simulink model "windEmulatorStep4"  (R2022b)
settings: Solver=ode4  StartTime=0.0  StopTime=inf  FixedStep=Ts  RelTol=1e-3
values from neighbouring files (symbols this model uses):
  A = 1.0    (= 1)    [initStep4.m]
  absEncoderCountsToRad = 1/2^20*2*pi    (= 5.99211245268e-06)    [initStep4.m]
  acs800DcBusVoltsScaling = 1    [initStep4.m]
  acs800FreqScaling = 1/100    (= 0.01)    [initStep4.m]
  acs800PowerScaling = Gen_PowerScaling    (= 14.9109)    [initStep4.m]
  acs800SpeedNomEng = 1500    [initStep4.m]
  acs800SpeedNomFb = 20000    [initStep4.m]
  acs800SpeedScaling = 1500/20000    (= 0.075)    [initStep4.m]
  acs800TempScaling = 1/10    (= 0.1)    [initStep4.m]
  acs800TorqueNomEng = 100    [initStep4.m]
  acs800TorqueNomFb = 10000    [initStep4.m]
  acs800TorqueScaling = acs800TorqueRating/10000    (= 0.008035933)    [initStep4.m]
  acs880FreqScaling = 60/20000    (= 0.003)    [initStep4.m]
  acs880MotorCurrentScaling = 100/10000    (= 0.01)    [initStep4.m]
  acs880MotorVoltsScaling = 1    [initStep4.m]
  acs880PowerScaling = 100*hp2W/10000    (= 7.457)    [initStep4.m]
  acs880RatedTorque = 80.494    [initStep4.m]
  acs880RateLimFalling = -10000    [initStep4.m]
  acs880RateLimRising = 10000    [initStep4.m]
  acs880SetpointLimLower = -0.975*acs880RatedTorque    (= -78.48165)    [initStep4.m]
  acs880SetpointLimUpper = 0.975*acs880RatedTorque    (= 78.48165)    [initStep4.m]
  acs880SpeedPILimLo = -0.975*acs880RatedTorque    (= -78.48165)    [initStep4.m]
  acs880SpeedPILimUp = 0.975*acs880RatedTorque    (= 78.48165)    [initStep4.m]
  acs880SpeedScaling = 2000/20000    (= 0.1)    [initStep4.m]
  acs880TorqueFieldbusScale = 10000    [initStep4.m]
  acs880TorqueScaling = acs880RatedTorque/acs880TorqueFieldbusScale    (= 0.0080494)    [initStep4.m]
  acs880TorqueSetpointScaling = 100    [initStep4.m]
  bar2pa = 1e5    (= 100000)    [initStep4.m]
  belowMinPGain = 1/200    (= 0.005)    [initStep4.m]
  ctrlModeTorque = logical(true)    [initStep4.m]
  deadBandController = boolean(true)    [initStep4.m]
  deadbandTorqueSlewRate = 300    [initStep4.m]
  Dm_max = 40    [initStep4.m]
  EffMechMax = 0.93    [initStep4.m]
  EffMechMin = 0.79    [initStep4.m]
  FactorEff = psi2pa*cc2m3*(1/rev2rad)    (= 0.00109733470463)    [initStep4.m]
  fromFileSpeedSlewRate = 250    [initStep4.m]
  fromFileTorqueSlewRate = 25    [initStep4.m]
  futekTorqueScale = -1/(2^31)*10/5*100    (= -9.31322574615e-08)    [initStep4.m]
  genMaxTorque = 0.975*acs880RatedTorque    (= 78.48165)    [initStep4.m]
  hbmCtScale = 1/1.5    (= 0.666666666667)    [initStep4.m]
  lpm2m3ps = 1/m3ps2lpm    (= 1.66666666667e-05)    [initStep4.m]
  minPressureRef_psi = 1000    [initStep4.m]
  minTorqueRef_Nm = (minPressureRef_psi*psi2pa)*(Dm_max*cc2m3*(1/rev2rad))    (= 43.8933881851)    [initStep4.m]
  nPreDrop = 2900    [initStep4.m]
  nPreDropMin = 725    [initStep4.m]
  psi2bar = 1/bar2psi    (= 0.0689475729318)    [initStep4.m]
  radps2rpm = 1/rpm2radps    (= 9.54929658551)    [initStep4.m]
  rpm2radps = 2*pi/60    (= 0.10471975512)    [initStep4.m]
  sidDataCaseCounter = sidData.experimentData.count    [initStep4.m]
  sidDataSpeed_rpm = sidData.experimentData.wShaft_rpm    [initStep4.m]
  sidDataTorque_Nm = sidData.experimentData.torqueShaft_Nm    [initStep4.m]
  StatusWord = bitset(StatusWord,16)    [VFD_StatusWord.m]
  T = 4    [initStep4.m]
  targetOmega = 2000/60*2*pi    (= 209.439510239)    [initStep4.m]
  TorqueLoadMax = 75    [initStep4.m]
  Ts = 1/250    (= 0.004)    [initStep4.m]
undefined symbols (not defined in the file or in its folder): absEncoderCounts, absEncoderPosition_rad, absEncoderSpeed_rpm, absEncoderStatus1, absEncoderStatus2, absEncoderTurns, acs800CtrlStruct, acs800SignalStruct, acs800Torque_Nm, acs800TorqueSetpoint_Nm, acs880CtrlStruct, acs880SignalStruct, acs880SpeedSetpoint_rpm, acs880Torque_Nm, ctrlSignal1, ctrlSignal2, ctrlWord, dcBusVoltage_V, DiscIntNeverNeededParam, excForce_N, excShaftSpeed_rpm, excShaftTorque_Nm, expCtrlStruct, expType, expTypeEnum, frequency_Hz, fromFileCaseCounter, genPumpFlow_lpm, genShaftSpeed_rpm, genSpeedActual, genTorqueCmd_Nm, hbmPowerStruct, hmOutputShafTorque_Nm, hptoCtrlStruct, hptoSignalStruct, invPowerStruct, motorCurrent_A, motorSpeed_rpm, motorTorque_Nm, motorVoltage_V, pressure_bar, PressureControl, ramp, resetHilIntegrator, resetSidIntegrator, runCounter, runHil, runSid, shaftPower_W, shaftSignalStruct, sidCtrlStruct, sidInfoStruct, sidType, sidTypeEnum, SpeedControl, speedCtrlReset, speedRef_rpm, state, statusWord, stepCounter ... (+6)
libraries: slrealtimeethercatlib x118, fl_lib x26, nesl_utility x17, slrealtimeloglib x13, sh_lib x9, dspstat3 x5, simulink_extras x4, slpidlib x3, cstblocks x3, dspindex x3, simulink x2
(part 5 of 5)

== system windEmulatorStep4/hptoSim/hptoModel/ControlAlgorithm/PressureAbovePmin/SpeedControl1/Subsystem ==
  shaftSpeedRef : Inport
  shaftSpeedMotor : Inport  Port=2
  Reset : Inport  Port=3
  Constant : Constant  Value=genMaxTorque
  Constant1 : Constant  Value=-genMaxTorque
  Gain2 : Gain  Gain=-1
  PID Controller : slpidlib/PID Controller  Controller=PID  Form=Parallel  TimeDomain=Discrete-time  UseExternalTs=off  SampleTime=-1  IntegratorMethod=Forward Euler  FilterMethod=Forward Euler  ControllerParametersSource=internal  P=SpeedControl.PG  I=SpeedControl.IG  UseKiTs=off  D=0  N=100  UseFilter=on  TunerSelectOption=Transfer Function Based (PID Tuner App)  InitialConditionSource=internal  InitialConditionForIntegrator=0  InitialConditionForFilter=0  DifferentiatorICPrevScaledInput=0  ExternalReset=level  TrackingMode=off  Kt=1  LimitOutput=on  SatLimitsSource=external  UpperSaturationLimit=inf  LowerSaturationLimit=-inf  LinearizeAsGain=on  AntiWindupMode=none  Kb=1  LimitIntegrator=off  UpperIntegratorSaturationLimit=inf  LowerIntegratorSaturationLimit=-inf  POutMin=[]  POutMax=[]  IOutMin=[]  IOutMax=[]  DOutMin=[]  DOutMax=[]  NOutMin=[]  NOutMax=[]  SumOutMin=[]  SumOutMax=[]  SaturationOutMin=[]  SaturationOutMax=[]  PParamMin=[]  PParamMax=[]  IParamMin=[]  IParamMax=[]  DParamMin=[]  DParamMax=[]  NParamMin=[]  NParamMax=[]  KbParamMin=[]  KbParamMax=[]  KtParamMin=[]  KtParamMax=[]  KbOutMin=[]  KbOutMax=[]  KtOutMin=[]  KtOutMax=[]  IntegratorOutMin=[]  IntegratorOutMax=[]  FilterOutMin=[]  FilterOutMax=[]  SumI1OutMin=[]  SumI1OutMax=[]  SumI2OutMin=[]  SumI2OutMax=[]  SumI3OutMin=[]  SumI3OutMax=[]  SumI4OutMin=[]  SumI4OutMax=[]  SumDOutMin=[]  SumDOutMax=[]  DifferentiatorOutMin=[]  DifferentiatorOutMax=[]  FilterDiffOutCoefMin=[]  FilterDiffOutCoefMax=[]  ReciprocalOutMin=[]  ReciprocalOutMax=[]  SumDenOutMin=[]  SumDenOutMax=[]  SumNumOutMin=[]  SumNumOutMax=[]  DivideOutMin=[]  DivideOutMax=[]  UdiffTsProdOutMin=[]  UdiffTsProdOutMax=[]  NTsProdOutMin=[]  NTsProdOutMax=[]  UintegralTsProdOutMin=[]  UintegralTsProdOutMax=[]  UngainTsProdOutMin=[]  UngainTsProdOutMax=[]  ClampingZeroOutDataTypeStr=Inherit: Inherit via back propagation  ClampingZeroOutMin=[]  ClampingZeroOutMax=[]  FilterDenConstantOutDataTypeStr=Inherit: Inherit via back propagation  FilterDenConstantOutMin=[]  FilterDenConstantOutMax=[]  PCopyOutDataTypeStr=Inherit: Inherit via back propagation  PCopyOutMin=[]  PCopyOutMax=[]  NCopyOutDataTypeStr=Inherit: Inherit via back propagation  NCopyOutMin=[]  NCopyOutMax=[]  IntegratorContinuousStateAttributes=''  IntegratorStateMustResolveToSignalObject=off  IntegratorRTWStateStorageClass=Auto  FilterContinuousStateAttributes=''  FilterStateMustResolveToSignalObject=off  FilterRTWStateStorageClass=Auto  ParallelPVariant=InternalParameters  IdealPVariant=Disabled  IVariant=InternalParameters  DVariant=InternalParameters  IntegratorVariant=Discrete  SatVariant=External  AWVariant=Passthrough  PCopyVariant=Disabled  TRVariant=Disabled  FdbkBlocksVariant=Forward  IdealPFdbkVariant=Disabled  SatFdbkVariant=Disabled  DerivativeFilterVariant=ForwardEulerFilter  NVariant=InternalParameters  NCopyVariant=Disabled  FilterICVariant=InternalICsFilter  IntegratorICVariant=InternalICs  ExternalResetVariant=ExternalReset  TRSumVariant=Passthrough  SumFdbkVariant=Disabled  SumVariant=Sum_PID  TsampFilterVariant=InternalTs  TsampNgainVariant=Passthrough  TsampIntegralVariant=Passthrough  ExternalSaturationOutDataTypeStr=Inherit: Same as second input
  Sum : Sum  Inputs=|-+
  ContolTorque_Nm : Outport
  wires:
  shaftSpeedRef/1 -> Sum/1
  PID Controller/1 -> Gain2/1
  Reset/1 -> PID Controller/2
  Constant/1 -> PID Controller/3
  Gain2/1 -> ContolTorque_Nm/1  "ContolTorque"
  Sum/1 -> PID Controller/1  "wError"
  Constant1/1 -> PID Controller/4
  shaftSpeedMotor/1 -> Sum/2

== system windEmulatorStep4/hptoSim/hptoModel/ControlAlgorithm/PressureAbovePmin/SpeedControl1/Subsystem1 ==
  ShaftSpeed : Inport
  ShaftSpeedRefMax : Inport  Port=2
  ShaftSpeedRefMin : Inport  Port=3
  Add : Sum  Inputs=+-
  Add1 : Sum  Inputs=+-
  Constant1 : Constant  Value=0
  Gain : Gain  Gain=TorqueLoadMax
  Subsystem : Subsystem
  Subsystem1 : Subsystem
  Switch : Switch  Criteria=u2 > Threshold  SaturateOnIntegerOverflow=off  InputSameDT=off
  Switch1 : Switch  Criteria=u2 > Threshold  SaturateOnIntegerOverflow=off  InputSameDT=off
  ControlTorque_Nm : Outport
  wires:
  ShaftSpeedRefMax/1 -> Add/2, Subsystem/2(ShaftSpeedRef)
  ShaftSpeed/1 -> Add/1, Subsystem1/3(ShaftSpeed), Subsystem/3(ShaftSpeed), Add1/1
  Add/1 -> Switch/2, Subsystem/1(Error)
  ShaftSpeedRefMin/1 -> Add1/2, Subsystem1/2(ShaftSpeedRefMin)
  Subsystem/1(ControlSignal3) -> Switch/1
  Switch1/1 -> Switch/3
  Switch/1 -> Gain/1
  Gain/1 -> ControlTorque_Nm/1
  Constant1/1 -> Switch1/1
  Add1/1 -> Switch1/2, Subsystem1/1(Error)
  Subsystem1/1(ControlSignal3) -> Switch1/3

== system windEmulatorStep4/hptoSim/hptoModel/ControlAlgorithm/PressureBelowPmin/SpeedControl1/Subsystem ==
  shaftSpeedRef : Inport
  shaftSpeedMotor : Inport  Port=2
  Reset : Inport  Port=3
  Constant : Constant  Value=genMaxTorque
  Constant1 : Constant  Value=-genMaxTorque
  Gain2 : Gain  Gain=-1
  PID Controller : slpidlib/PID Controller  Controller=PID  Form=Parallel  TimeDomain=Discrete-time  UseExternalTs=off  SampleTime=-1  IntegratorMethod=Forward Euler  FilterMethod=Forward Euler  ControllerParametersSource=internal  P=SpeedControl.PG  I=SpeedControl.IG  UseKiTs=off  D=0  N=100  UseFilter=on  TunerSelectOption=Transfer Function Based (PID Tuner App)  InitialConditionSource=internal  InitialConditionForIntegrator=0  InitialConditionForFilter=0  DifferentiatorICPrevScaledInput=0  ExternalReset=level  TrackingMode=off  Kt=1  LimitOutput=on  SatLimitsSource=external  UpperSaturationLimit=inf  LowerSaturationLimit=-inf  LinearizeAsGain=on  AntiWindupMode=none  Kb=1  LimitIntegrator=off  UpperIntegratorSaturationLimit=inf  LowerIntegratorSaturationLimit=-inf  POutMin=[]  POutMax=[]  IOutMin=[]  IOutMax=[]  DOutMin=[]  DOutMax=[]  NOutMin=[]  NOutMax=[]  SumOutMin=[]  SumOutMax=[]  SaturationOutMin=[]  SaturationOutMax=[]  PParamMin=[]  PParamMax=[]  IParamMin=[]  IParamMax=[]  DParamMin=[]  DParamMax=[]  NParamMin=[]  NParamMax=[]  KbParamMin=[]  KbParamMax=[]  KtParamMin=[]  KtParamMax=[]  KbOutMin=[]  KbOutMax=[]  KtOutMin=[]  KtOutMax=[]  IntegratorOutMin=[]  IntegratorOutMax=[]  FilterOutMin=[]  FilterOutMax=[]  SumI1OutMin=[]  SumI1OutMax=[]  SumI2OutMin=[]  SumI2OutMax=[]  SumI3OutMin=[]  SumI3OutMax=[]  SumI4OutMin=[]  SumI4OutMax=[]  SumDOutMin=[]  SumDOutMax=[]  DifferentiatorOutMin=[]  DifferentiatorOutMax=[]  FilterDiffOutCoefMin=[]  FilterDiffOutCoefMax=[]  ReciprocalOutMin=[]  ReciprocalOutMax=[]  SumDenOutMin=[]  SumDenOutMax=[]  SumNumOutMin=[]  SumNumOutMax=[]  DivideOutMin=[]  DivideOutMax=[]  UdiffTsProdOutMin=[]  UdiffTsProdOutMax=[]  NTsProdOutMin=[]  NTsProdOutMax=[]  UintegralTsProdOutMin=[]  UintegralTsProdOutMax=[]  UngainTsProdOutMin=[]  UngainTsProdOutMax=[]  ClampingZeroOutDataTypeStr=Inherit: Inherit via back propagation  ClampingZeroOutMin=[]  ClampingZeroOutMax=[]  FilterDenConstantOutDataTypeStr=Inherit: Inherit via back propagation  FilterDenConstantOutMin=[]  FilterDenConstantOutMax=[]  PCopyOutDataTypeStr=Inherit: Inherit via back propagation  PCopyOutMin=[]  PCopyOutMax=[]  NCopyOutDataTypeStr=Inherit: Inherit via back propagation  NCopyOutMin=[]  NCopyOutMax=[]  IntegratorContinuousStateAttributes=''  IntegratorStateMustResolveToSignalObject=off  IntegratorRTWStateStorageClass=Auto  FilterContinuousStateAttributes=''  FilterStateMustResolveToSignalObject=off  FilterRTWStateStorageClass=Auto  ParallelPVariant=InternalParameters  IdealPVariant=Disabled  IVariant=InternalParameters  DVariant=InternalParameters  IntegratorVariant=Discrete  SatVariant=External  AWVariant=Passthrough  PCopyVariant=Disabled  TRVariant=Disabled  FdbkBlocksVariant=Forward  IdealPFdbkVariant=Disabled  SatFdbkVariant=Disabled  DerivativeFilterVariant=ForwardEulerFilter  NVariant=InternalParameters  NCopyVariant=Disabled  FilterICVariant=InternalICsFilter  IntegratorICVariant=InternalICs  ExternalResetVariant=ExternalReset  TRSumVariant=Passthrough  SumFdbkVariant=Disabled  SumVariant=Sum_PID  TsampFilterVariant=InternalTs  TsampNgainVariant=Passthrough  TsampIntegralVariant=Passthrough  ExternalSaturationOutDataTypeStr=Inherit: Same as second input
  Sum : Sum  Inputs=|-+
  ContolTorque : Outport
  wires:
  shaftSpeedRef/1 -> Sum/1
  PID Controller/1 -> Gain2/1
  Reset/1 -> PID Controller/2
  Constant/1 -> PID Controller/3
  Gain2/1 -> ContolTorque/1  "ContolTorque"
  Sum/1 -> PID Controller/1  "wError"
  Constant1/1 -> PID Controller/4
  shaftSpeedMotor/1 -> Sum/2

== system windEmulatorStep4/hptoSim/hptoModel/ControlAlgorithm/PressureBelowPmin/SpeedControl1/Subsystem1 ==
  ShaftSpeed : Inport
  ShaftSpeedRefMax : Inport  Port=2
  ShaftSpeedRefMin : Inport  Port=3
  Add : Sum  Inputs=+-
  Add1 : Sum  Inputs=+-
  Constant1 : Constant  Value=0
  Gain : Gain  Gain=TorqueLoadMax
  Subsystem : Subsystem
  Subsystem1 : Subsystem
  Switch : Switch  Criteria=u2 > Threshold  SaturateOnIntegerOverflow=off  InputSameDT=off
  Switch1 : Switch  Criteria=u2 > Threshold  SaturateOnIntegerOverflow=off  InputSameDT=off
  ControlTorque : Outport
  wires:
  ShaftSpeedRefMax/1 -> Add/2, Subsystem/2(ShaftSpeedRef)
  ShaftSpeed/1 -> Add/1, Subsystem1/3(ShaftSpeed), Subsystem/3(ShaftSpeed), Add1/1
  Add/1 -> Switch/2, Subsystem/1(Error)
  ShaftSpeedRefMin/1 -> Add1/2, Subsystem1/2(ShaftSpeedRefMin)
  Subsystem/1(ControlSignal3) -> Switch/1
  Switch1/1 -> Switch/3
  Switch/1 -> Gain/1
  Gain/1 -> ControlTorque/1
  Constant1/1 -> Switch1/1
  Add1/1 -> Switch1/2, Subsystem1/1(Error)
  Subsystem1/1(ControlSignal3) -> Switch1/3

== system windEmulatorStep4/hptoSim/hptoModel/ControlAlgorithm/PressureAbovePmin/SpeedControl1/Subsystem1/Subsystem ==
  Error : Inport
  ShaftSpeedRef : Inport  Port=2
  ShaftSpeed : Inport  Port=3
  Constant : Constant  Value=0  OutDataTypeStr=boolean
  Constant1 : Constant  Value=-SpeedControl.PG
  Product : Product
  Relational Operator : RelationalOperator  Operator=<=  RndMeth=Simplest  InputSameDT=off
  S-R Flip-Flop : simulink_extras/Flip Flops/S-R Flip-Flop  initial_condition=0
  Saturation : Saturate  UpperLimit=0  LowerLimit=-1
  Switch : Switch  Criteria=u2 > Threshold  OutDataTypeStr=double  SaturateOnIntegerOverflow=off  InputSameDT=off
  Terminator : Terminator
  ControlSignal3 : Outport
  wires:
  ShaftSpeedRef/1 -> Relational Operator/1  "ShaftSpeedRef"
  S-R Flip-Flop/2 -> Terminator/1
  Error/1 -> Product/2
  Saturation/1 -> Switch/1
  Switch/1 -> ControlSignal3/1  "ControlSignal3"
  Product/1 -> Saturation/1, Switch/3  "ControlSignal31"
  Relational Operator/1 -> S-R Flip-Flop/1
  S-R Flip-Flop/1 -> Switch/2
  Constant/1 -> S-R Flip-Flop/2
  ShaftSpeed/1 -> Relational Operator/2
  Constant1/1 -> Product/1

== system windEmulatorStep4/hptoSim/hptoModel/ControlAlgorithm/PressureAbovePmin/SpeedControl1/Subsystem1/Subsystem1 ==
  Error : Inport
  ShaftSpeedRefMin : Inport  Port=2
  ShaftSpeed : Inport  Port=3
  Constant : Constant  Value=0  OutDataTypeStr=boolean
  Constant1 : Constant  Value=-belowMinPGain
  Product : Product
  Relational Operator : RelationalOperator  RndMeth=Simplest  InputSameDT=off
  S-R Flip-Flop : simulink_extras/Flip Flops/S-R Flip-Flop  initial_condition=0
  Saturation : Saturate  UpperLimit=1  LowerLimit=0
  Switch : Switch  Criteria=u2 > Threshold  OutDataTypeStr=double  SaturateOnIntegerOverflow=off  InputSameDT=off
  Terminator : Terminator
  ControlSignal3 : Outport
  wires:
  ShaftSpeedRefMin/1 -> Relational Operator/1  "ShaftSpeedRefMin"
  S-R Flip-Flop/2 -> Terminator/1
  Error/1 -> Product/2
  Saturation/1 -> Switch/1
  Switch/1 -> ControlSignal3/1  "ControlSignal3"
  Product/1 -> Saturation/1, Switch/3  "ControlSignal31"
  Relational Operator/1 -> S-R Flip-Flop/1
  S-R Flip-Flop/1 -> Switch/2
  Constant/1 -> S-R Flip-Flop/2
  ShaftSpeed/1 -> Relational Operator/2
  Constant1/1 -> Product/1

== system windEmulatorStep4/hptoSim/hptoModel/ControlAlgorithm/PressureBelowPmin/SpeedControl1/Subsystem1/Subsystem ==
  Error : Inport
  ShaftSpeedRef : Inport  Port=2
  ShaftSpeed : Inport  Port=3
  Constant : Constant  Value=0  OutDataTypeStr=boolean
  Constant1 : Constant  Value=-SpeedControl.PG
  Product : Product
  Relational Operator : RelationalOperator  Operator=<=  RndMeth=Simplest  InputSameDT=off
  S-R Flip-Flop : simulink_extras/Flip Flops/S-R Flip-Flop  initial_condition=0
  Saturation : Saturate  UpperLimit=0  LowerLimit=-1
  Switch : Switch  Criteria=u2 > Threshold  OutDataTypeStr=double  SaturateOnIntegerOverflow=off  InputSameDT=off
  Terminator : Terminator
  ControlSignal3 : Outport
  wires:
  ShaftSpeedRef/1 -> Relational Operator/1  "ShaftSpeedRef"
  S-R Flip-Flop/2 -> Terminator/1
  Error/1 -> Product/2
  Saturation/1 -> Switch/1
  Switch/1 -> ControlSignal3/1  "ControlSignal3"
  Product/1 -> Saturation/1, Switch/3  "ControlSignal31"
  Relational Operator/1 -> S-R Flip-Flop/1
  S-R Flip-Flop/1 -> Switch/2
  Constant/1 -> S-R Flip-Flop/2
  ShaftSpeed/1 -> Relational Operator/2
  Constant1/1 -> Product/1

== system windEmulatorStep4/hptoSim/hptoModel/ControlAlgorithm/PressureBelowPmin/SpeedControl1/Subsystem1/Subsystem1 ==
  Error : Inport
  ShaftSpeedRefMin : Inport  Port=2
  ShaftSpeed : Inport  Port=3
  Constant : Constant  Value=0  OutDataTypeStr=boolean
  Constant1 : Constant  Value=-belowMinPGain
  Product : Product
  Relational Operator : RelationalOperator  RndMeth=Simplest  InputSameDT=off
  S-R Flip-Flop : simulink_extras/Flip Flops/S-R Flip-Flop  initial_condition=0
  Saturation : Saturate  UpperLimit=1  LowerLimit=0
  Switch : Switch  Criteria=u2 > Threshold  OutDataTypeStr=double  SaturateOnIntegerOverflow=off  InputSameDT=off
  Terminator : Terminator
  ControlSignal3 : Outport
  wires:
  ShaftSpeedRefMin/1 -> Relational Operator/1  "ShaftSpeedRefMin"
  S-R Flip-Flop/2 -> Terminator/1
  Error/1 -> Product/2
  Saturation/1 -> Switch/1
  Switch/1 -> ControlSignal3/1  "ControlSignal3"
  Product/1 -> Saturation/1, Switch/3  "ControlSignal31"
  Relational Operator/1 -> S-R Flip-Flop/1
  S-R Flip-Flop/1 -> Switch/2
  Constant/1 -> S-R Flip-Flop/2
  ShaftSpeed/1 -> Relational Operator/2
  Constant1/1 -> Product/1

== matlab function windEmulatorStep4/fileAndUI/acs880SignalsUI/statusWordDetail/Parse Status Word ==
  data: StatusWord input; rdy_on output; rdy_run output; rdy_ref output; tripped output; off2 output; off3 output; swc_on_inhib output; alarm output; at_setpoint output; remote output; above_limit output; ext_ctrl_loc output; ext_run_enable output; msw_b13 output; msw_b14 output; comm_err output
function [rdy_on,rdy_run,rdy_ref,tripped,off2,off3,swc_on_inhib,alarm,...
    at_setpoint,remote,above_limit,ext_ctrl_loc,ext_run_enable,...
    msw_b13,msw_b14,comm_err]  = fcn(StatusWord)

SW = VFD_StatusWord(StatusWord);
rdy_on = SW.RDY_ON;
rdy_run = SW.RDY_RUN;
rdy_ref = SW.RDY_REF;
tripped = SW.TRIPPED;
off2 = SW.OFF_2_STA;
off3 = SW.OFF_3_STA;
swc_on_inhib = SW.SWC_ON_INHIB;
alarm = SW.ALARM;
at_setpoint = SW.AT_SETPOINT;
remote = SW.REMOTE;
above_limit = SW.ABOVE_LIMIT;
ext_ctrl_loc = SW.EXT_CTRL_LOC;
ext_run_enable = SW.EXT_RUN_ENABLE;
msw_b13 = SW.MSW_B13;
msw_b14 = SW.MSW_B14;
comm_err = SW.COMM_ERR;

== stateflow chart windEmulatorStep4/expCtrl/FexcRamp ==
  state init
    entry:
    runCounter = uint32(0);
    stepCounter = uint32(1);
    ramp=0;
    rampLast=0;
    time = 0; rampUpTime = 0; runTime = 0;
    resetHilIntegrator = true;
    resetSidIntegrator = true;
  state idle
    during:
    ramp=0;
    rampLast=0;
    stepCounter = uint32(1); % one-based index for array
    time = 0; rampUpTime = 0; runTime = 0;
    resetHilIntegrator = true;
    resetSidIntegrator = true;
  state rampup
    entry:
    runCounter = runCounter + uint32(1);
    resetHilIntegrator = ~(expType == expTypeEnum.hil);
    resetSidIntegrator = ~(expType == expTypeEnum.sid);
    during:
    ramp=min(1,elapsed('sec')/rampTime);
    stepCounter = stepCounter + uint32(1);
    rampLast = ramp;
    rampUpTime = elapsed('sec');
    time = rampUpTime;
  state runing
    during:
    ramp=1
    rampLast = ramp
    runTime = elapsed('sec');
    time = rampUpTime + runTime;
    stepCounter = stepCounter + uint32(1);
    resetHilIntegrator = ~(expType == expTypeEnum.hil);
    resetSidIntegrator = ~(expType == expTypeEnum.sid);
  state rampdown
    during:
    ramp=rampLast-max(0,elapsed('sec')/rampTime)
    time = rampUpTime + runTime + elapsed('sec');
    stepCounter = stepCounter + uint32(1);
    resetHilIntegrator = ~(expType == expTypeEnum.hil);
    resetSidIntegrator = ~(expType == expTypeEnum.sid);
  (default) -> init
  init -> idle
  rampdown -> idle : [ramp<=0]
  idle -> rampup : [startButton]
  rampup -> rampdown [order 1] : [stopButton]
  rampup -> runing [order 2] : [ramp>=1]
  runing -> rampdown : [stopButton || time >= expRunTime]
  data: expType input Enum: expTypeEnum; time output; ramp output; rampLast local; rampTime parameter; rampUpTime local; runTime local; runCounter output uint32; stepCounter output; startButton input; stopButton input; expRunTime input; resetHilIntegrator output boolean; resetSidIntegrator output boolean

== matlab function windEmulatorStep4/fileAndUI/acs800CtrlSignalsUI/ctrlWordDetail/parseCtrlWord ==
  data: ctrlWord input; off1Ctrl output; off2Ctrl output; off3Ctrl output; enableOperation output; rampOutZero output; rampHold output; rampInZero output; reset output; inching1 output; inching2 output; remoteCmd output; extCtrlLoc output
function [  off1Ctrl, ...
            off2Ctrl, ...
            off3Ctrl, ...
            enableOperation, ...
            rampOutZero, ...
            rampHold, ...
            rampInZero, ...
            reset, ...
            inching1, ...
            inching2, ...
            remoteCmd, ...
            extCtrlLoc] ...
              = fcn(ctrlWord)   

%TODO - should define position of each bit in init script
off1Ctrl = bitget(ctrlWord,1);
off2Ctrl = bitget(ctrlWord,2);
off3Ctrl = bitget(ctrlWord,3);
enableOperation = bitget(ctrlWord,4);
rampOutZero = bitget(ctrlWord,5);
rampHold = bitget(ctrlWord,6);
rampInZero = bitget(ctrlWord,7);
reset = bitget(ctrlWord,8);
inching1 = bitget(ctrlWord,9);
inching2 = bitget(ctrlWord,10);
remoteCmd = bitget(ctrlWord,11);
extCtrlLoc = bitget(ctrlWord,12);

== stateflow chart windEmulatorStep4/acs880Ctrl/ACS880Ramp ==
  state idle
    during:
    ramp=0
    rampLast=0
  state rampup
    during:
    ramp=min(1,elapsed('sec')/rampTime)
    rampLast = ramp
  state runing
    during:
    ramp=1
    rampLast = ramp
  state rampdown
    during:
    ramp=rampLast-max(0,elapsed('sec')/rampTime)
  (default) -> idle
  rampdown -> idle : [ramp<=0]
  idle -> rampup : [runButton]
  rampup -> rampdown [order 2] : [~runButton]
  rampup -> runing [order 1] : [ramp>=1]
  runing -> rampdown : [~runButton]
  data: ramp output; runButton input; rampLast local; rampTime parameter

== stateflow chart windEmulatorStep4/acs880Ctrl/ACS880FieldbusControl/ABB Fieldbus Control ==
  state UpdateStateMachine [parallel]
    during:
    swParseStatusWord();
    cwRESET = resetFault;
    settings: executionOrder=1
    state initialize
      entry:
      cwInitialize();
      state=abbStateEnum.init
    state notReadyToSwitchOn
      entry:
      cwOFF1_CONTROL=0;
      during:
      state=abbStateEnum.notReadyToSwitchOn
    state readyToSwitchOn
      entry:
      cwOFF1_CONTROL=0;
      during:
      state=abbStateEnum.readyToSwitchOn
    state operationDisabled
      entry:
      cwOFF1_CONTROL=1;
      during:
      state=abbStateEnum.operationDisabled
    state DelayOFF1
      during:
      state=abbStateEnum.delayOff1
    note: Note: probably best to introduce extra state here once swRdy_Run is true
    state operationEnabled
      entry:
      cwOFF1_CONTROL=1;
      cwENABLE_OPERATION=1;
      during:
      state=abbStateEnum.operationEnabled
      exit:
      cwENABLE_OPERATION=0;
    (default) -> initialize
    initialize -> notReadyToSwitchOn
    DelayOFF1 -> notReadyToSwitchOn : after(100,msec)
    notReadyToSwitchOn -> readyToSwitchOn : [swRDY_ON==1 && ...
        |  swWARNING==0]
    readyToSwitchOn -> operationDisabled : [powerUp && ...
        |  swREMOTE==1]
    operationDisabled -> DelayOFF1 [order 2] : [powerDown || ...
        | eStop || ...
        |  swTRIPPED==1 || ...
        |  swSWC_ON_INHIB==1 || ...
        |  swWARNING==1]
    operationEnabled -> DelayOFF1 [order 2] : [eStop || ...
        |  swTRIPPED==1 || ...
        |  swSWC_ON_INHIB==1 || ...
        |  swWARNING==1]
    operationDisabled -> operationEnabled [order 1] : [powerUp && ...
        | swRDY_RUN==1]
    operationEnabled -> operationDisabled [order 1] : [powerDown]
  state UpdateControlWord [parallel]
    during:
    cwBuildControlWord();
    settings: executionOrder=2
  data: powerUp input; powerDown input; resetFault input; eStop input; StatusWord input; swRDY_ON local; swRDY_RUN local; swRDY_REF local; swTRIPPED local; swOFF_2_STA local; swOFF_3_STA local; swSWC_ON_INHIB local; swAT_SETPOINT local; swEXT_RUN_ENABLE local; cwOFF2_CONTROL local; cwOFF3_CONTROL local; cwENABLE_OPERATION local; cwRAMP_OUT_ZERO local; cwRAMP_HOLD local; cwRAMP_IN_ZERO local; cwRESET local; cwREMOTE_CMD local; cwOFF1_CONTROL local; swEXT_CTRL_LOC local; swREMOTE local; ControlWord output uint16; swWARNING local; swABOVE_LIMIT local; swMSW_B13 local; swMSW_B14 local; swCOMM_ERR local; state output; cwEXT_CTRL_LOC input
  function cwInitialize:
    | function cwInitialize
    | cwOFF1_CONTROL = 0;
    | cwOFF2_CONTROL = 1;
    | cwOFF3_CONTROL = 1;
    | cwENABLE_OPERATION = 0;
    | cwRAMP_OUT_ZERO = 1;
    | cwRAMP_HOLD = 1;
    | cwRAMP_IN_ZERO = 1;
    | cwRESET = 0;
    | % cwINCHING_1 = 0;
    | % cwINCHING_2 = 0;
    | cwREMOTE_CMD = 1;
    | %cwEXT_CTRL_LOC = 0;
  function cwBuildControlWord:
    | function cwBuildControlWord
    | ControlWord = uint16(0);
    | if cwOFF1_CONTROL
    |     ControlWord = bitset(ControlWord,1);
    | end
    | if cwOFF2_CONTROL
    |     ControlWord = bitset(ControlWord,2);
    | end
    | if cwOFF3_CONTROL
    |     ControlWord = bitset(ControlWord,3);
    | end
    | if cwENABLE_OPERATION
    |     ControlWord = bitset(ControlWord,4);
    | end
    | if cwRAMP_OUT_ZERO
    |     ControlWord = bitset(ControlWord,5);
    | end
    | if cwRAMP_HOLD
    |     ControlWord = bitset(ControlWord,6);
    | end
    | if cwRAMP_IN_ZERO
    |     ControlWord = bitset(ControlWord,7);
    | end
    | if cwRESET
    |     ControlWord = bitset(ControlWord,8);
    | end
    | % if cwINCHING_1
    | %     ControlWord = bitset(ControlWord,9);
    | % end
    | % if cwINCHING_2
    | %     ControlWord = bitset(ControlWord,10);
    | % end
    | if cwREMOTE_CMD
    |     ControlWord = bitset(ControlWord,11);
    | end
    | if cwEXT_CTRL_LOC
    |     ControlWord = bitset(ControlWord,12);
    | end
  function swParseStatusWord:
    | function swParseStatusWord
    | sw = uint16(StatusWord);
    | swRDY_ON = 0;
    | swRDY_RUN = 0;
    | swRDY_REF = 0;
    | swTRIPPED = 0;
    | swOFF_2_STA = 0;
    | swOFF_3_STA = 0;
    | swSWC_ON_INHIB = 0;
    | swWARNING = 0;
    | swAT_SETPOINT = 0;
    | swREMOTE = 0;
    | swABOVE_LIMIT = 0;
    | swEXT_CTRL_LOC = 0;
    | swEXT_RUN_ENABLE = 0;
    | swMSW_B13 = 0;
    | swMSW_B14 = 0;
    | swCOMM_ERR = 0;
    | 
    | if (sw >= 2^15)
    |     swCOMM_ERR = 1;
    |     sw = sw - 2^15;
    | end
    | if (sw >= 2^14)
    |     swMSW_B14 = 1;
    |     sw = sw - 2^14;
    | end
    | if (sw >= 2^13)
    |     swMSW_B13 = 1;
    |     sw = sw - 2^13;
    | end
    | if (sw >= 2^12)
    |     swEXT_RUN_ENABLE = 1;
    |     sw = sw - 2^12;
    | end
    | if (sw >= 2^11)
    |     swEXT_CTRL_LOC = 1;
    |     sw = sw - 2^11;
    | end
    | if (sw >= 2^10)
    |     swABOVE_LIMIT = 1;
    |     sw = sw - 2^10;
    | end
    | if (sw >= 2^9)
    |     swREMOTE = 1;
    |     sw = sw - 2^9;
    | end
    | if (sw >= 2^8)
    |     swAT_SETPOINT = 1;
    |     sw = sw - 2^8;
    | end
    | if (sw >= 2^7)
    |     swWARNING = 1;
    |     sw = sw - 2^7;
    | end
    | if (sw >= 2^6)
    |     swSWC_ON_INHIB = 1;
    |     sw = sw - 2^6;
    | end
    | if (sw >= 2^5)
    |     swOFF_3_STA = 1;
    |     sw = sw - 2^5;
    | end
    | if (sw >= 2^4)
    |     swOFF_2_STA = 1;
    |     sw = sw - 2^4;
    | end
    | if (sw >= 2^3)
    |     swTRIPPED = 1;
    |     sw = sw - 2^3;
    | end
    | if (sw >= 2^2)
    |     swRDY_REF = 1;
    |     sw = sw - 2^2;
    | end
    | if (sw >= 2^1)
    |     swRDY_RUN = 1;
    |     sw = sw - 2^1;
    | end
    | if (sw >= 2^0)
    |     swRDY_ON = 1;
    |     sw = sw - 2^0;
    | end

== matlab function windEmulatorStep4/fileAndUI/acs880CtrlSignalsUI/ctrlWordDetail/parseCtrlWord ==
  data: ctrlWord input; off1Ctrl output; off2Ctrl output; off3Ctrl output; enableOperation output; rampOutZero output; rampHold output; rampInZero output; reset output; inching1 output; inching2 output; remoteCmd output; extCtrlLoc output
function [  off1Ctrl, ...
            off2Ctrl, ...
            off3Ctrl, ...
            enableOperation, ...
            rampOutZero, ...
            rampHold, ...
            rampInZero, ...
            reset, ...
            inching1, ...
            inching2, ...
            remoteCmd, ...
            extCtrlLoc] ...
              = fcn(ctrlWord)   

%TODO - should define position of each bit in init script
off1Ctrl = bitget(ctrlWord,1);
off2Ctrl = bitget(ctrlWord,2);
off3Ctrl = bitget(ctrlWord,3);
enableOperation = bitget(ctrlWord,4);
rampOutZero = bitget(ctrlWord,5);
rampHold = bitget(ctrlWord,6);
rampInZero = bitget(ctrlWord,7);
reset = bitget(ctrlWord,8);
inching1 = bitget(ctrlWord,9);
inching2 = bitget(ctrlWord,10);
remoteCmd = bitget(ctrlWord,11);
extCtrlLoc = bitget(ctrlWord,12);

== stateflow chart windEmulatorStep4/acs800Ctrl/ACS880FieldbusControl/ABB Fieldbus Control ==
  state UpdateStateMachine [parallel]
    during:
    swParseStatusWord();
    cwRESET = resetFault;
    settings: executionOrder=1
    state initialize
      entry:
      cwInitialize();
      state=abbStateEnum.init
    state notReadyToSwitchOn
      entry:
      cwOFF1_CONTROL=0;
      during:
      state=abbStateEnum.notReadyToSwitchOn
    state readyToSwitchOn
      entry:
      cwOFF1_CONTROL=0;
      during:
      state=abbStateEnum.readyToSwitchOn
    state operationDisabled
      entry:
      cwOFF1_CONTROL=1;
      during:
      state=abbStateEnum.operationDisabled
    state DelayOFF1
      during:
      state=abbStateEnum.delayOff1
    state operationEnabled
      entry:
      cwOFF1_CONTROL=1;
      cwENABLE_OPERATION=1;
      during:
      state=abbStateEnum.operationEnabled
      exit:
      cwENABLE_OPERATION=0;
    (default) -> initialize
    initialize -> notReadyToSwitchOn
    DelayOFF1 -> notReadyToSwitchOn : after(100,msec)
    notReadyToSwitchOn -> readyToSwitchOn : [swRDY_ON==1 && ...
        |  swWARNING==0]
    readyToSwitchOn -> operationDisabled : [powerUp && ...
        |  swREMOTE==1]
    operationDisabled -> DelayOFF1 [order 2] : [powerDown || ...
        | eStop || ...
        |  swTRIPPED==1 || ...
        |  swSWC_ON_INHIB==1 || ...
        |  swWARNING==1]
    operationEnabled -> DelayOFF1 [order 2] : [eStop || ...
        |  swTRIPPED==1 || ...
        |  swSWC_ON_INHIB==1]
    operationDisabled -> operationEnabled [order 1] : [powerUp && ...
        | swRDY_RUN==1]
    operationEnabled -> operationDisabled [order 1] : [powerDown]
  state UpdateControlWord [parallel]
    during:
    cwBuildControlWord();
    settings: executionOrder=2
  data: powerUp input; powerDown input; resetFault input; eStop input; StatusWord input; swRDY_ON local; swRDY_RUN local; swRDY_REF local; swTRIPPED local; swOFF_2_STA local; swOFF_3_STA local; swSWC_ON_INHIB local; swAT_SETPOINT local; swEXT_RUN_ENABLE local; cwOFF2_CONTROL local; cwOFF3_CONTROL local; cwENABLE_OPERATION local; cwRAMP_OUT_ZERO local; cwRAMP_HOLD local; cwRAMP_IN_ZERO local; cwRESET local; cwREMOTE_CMD local; cwOFF1_CONTROL local; swEXT_CTRL_LOC local; swREMOTE local; ControlWord output uint16; swWARNING local; swABOVE_LIMIT local; swMSW_B13 local; swMSW_B14 local; swCOMM_ERR local; state output; cwEXT_CTRL_LOC input
  function cwInitialize:
    | function cwInitialize
    | cwOFF1_CONTROL = 0;
    | cwOFF2_CONTROL = 1;
    | cwOFF3_CONTROL = 1;
    | cwENABLE_OPERATION = 0;
    | cwRAMP_OUT_ZERO = 1;
    | cwRAMP_HOLD = 1;
    | cwRAMP_IN_ZERO = 1;
    | cwRESET = 0;
    | % cwINCHING_1 = 0;
    | % cwINCHING_2 = 0;
    | cwREMOTE_CMD = 1;
    | %cwEXT_CTRL_LOC = 0;
  function cwBuildControlWord:
    | function cwBuildControlWord
    | ControlWord = uint16(0);
    | if cwOFF1_CONTROL
    |     ControlWord = bitset(ControlWord,1);
    | end
    | if cwOFF2_CONTROL
    |     ControlWord = bitset(ControlWord,2);
    | end
    | if cwOFF3_CONTROL
    |     ControlWord = bitset(ControlWord,3);
    | end
    | if cwENABLE_OPERATION
    |     ControlWord = bitset(ControlWord,4);
    | end
    | if cwRAMP_OUT_ZERO
    |     ControlWord = bitset(ControlWord,5);
    | end
    | if cwRAMP_HOLD
    |     ControlWord = bitset(ControlWord,6);
    | end
    | if cwRAMP_IN_ZERO
    |     ControlWord = bitset(ControlWord,7);
    | end
    | if cwRESET
    |     ControlWord = bitset(ControlWord,8);
    | end
    | % if cwINCHING_1
    | %     ControlWord = bitset(ControlWord,9);
    | % end
    | % if cwINCHING_2
    | %     ControlWord = bitset(ControlWord,10);
    | % end
    | if cwREMOTE_CMD
    |     ControlWord = bitset(ControlWord,11);
    | end
    | if cwEXT_CTRL_LOC
    |     ControlWord = bitset(ControlWord,12);
    | end
  function swParseStatusWord:
    | function swParseStatusWord
    | sw = uint16(StatusWord);
    | swRDY_ON = 0;
    | swRDY_RUN = 0;
    | swRDY_REF = 0;
    | swTRIPPED = 0;
    | swOFF_2_STA = 0;
    | swOFF_3_STA = 0;
    | swSWC_ON_INHIB = 0;
    | swWARNING = 0;
    | swAT_SETPOINT = 0;
    | swREMOTE = 0;
    | swABOVE_LIMIT = 0;
    | swEXT_CTRL_LOC = 0;
    | swEXT_RUN_ENABLE = 0;
    | swMSW_B13 = 0;
    | swMSW_B14 = 0;
    | swCOMM_ERR = 0;
    | 
    | if (sw >= 2^15)
    |     swCOMM_ERR = 1;
    |     sw = sw - 2^15;
    | end
    | if (sw >= 2^14)
    |     swMSW_B14 = 1;
    |     sw = sw - 2^14;
    | end
    | if (sw >= 2^13)
    |     swMSW_B13 = 1;
    |     sw = sw - 2^13;
    | end
    | if (sw >= 2^12)
    |     swEXT_RUN_ENABLE = 1;
    |     sw = sw - 2^12;
    | end
    | if (sw >= 2^11)
    |     swEXT_CTRL_LOC = 1;
    |     sw = sw - 2^11;
    | end
    | if (sw >= 2^10)
    |     swABOVE_LIMIT = 1;
    |     sw = sw - 2^10;
    | end
    | if (sw >= 2^9)
    |     swREMOTE = 1;
    |     sw = sw - 2^9;
    | end
    | if (sw >= 2^8)
    |     swAT_SETPOINT = 1;
    |     sw = sw - 2^8;
    | end
    | if (sw >= 2^7)
    |     swWARNING = 1;
    |     sw = sw - 2^7;
    | end
    | if (sw >= 2^6)
    |     swSWC_ON_INHIB = 1;
    |     sw = sw - 2^6;
    | end
    | if (sw >= 2^5)
    |     swOFF_3_STA = 1;
    |     sw = sw - 2^5;
    | end
    | if (sw >= 2^4)
    |     swOFF_2_STA = 1;
    |     sw = sw - 2^4;
    | end
    | if (sw >= 2^3)
    |     swTRIPPED = 1;
    |     sw = sw - 2^3;
    | end
    | if (sw >= 2^2)
    |     swRDY_REF = 1;
    |     sw = sw - 2^2;
    | end
    | if (sw >= 2^1)
    |     swRDY_RUN = 1;
    |     sw = sw - 2^1;
    | end
    | if (sw >= 2^0)
    |     swRDY_ON = 1;
    |     sw = sw - 2^0;
    | end

== matlab function windEmulatorStep4/fileAndUI/acs800SignalsUI/statusWordDetail/Parse Status Word ==
  data: StatusWord input; rdy_on output; rdy_run output; rdy_ref output; tripped output; off2 output; off3 output; swc_on_inhib output; alarm output; at_setpoint output; remote output; above_limit output; ext_ctrl_loc output; ext_run_enable output; msw_b13 output; msw_b14 output; comm_err output
function [rdy_on,rdy_run,rdy_ref,tripped,off2,off3,swc_on_inhib,alarm,...
    at_setpoint,remote,above_limit,ext_ctrl_loc,ext_run_enable,...
    msw_b13,msw_b14,comm_err]  = fcn(StatusWord)

SW = VFD_StatusWord(StatusWord);
rdy_on = SW.RDY_ON;
rdy_run = SW.RDY_RUN;
rdy_ref = SW.RDY_REF;
tripped = SW.TRIPPED;
off2 = SW.OFF_2_STA;
off3 = SW.OFF_3_STA;
swc_on_inhib = SW.SWC_ON_INHIB;
alarm = SW.ALARM;
at_setpoint = SW.AT_SETPOINT;
remote = SW.REMOTE;
above_limit = SW.ABOVE_LIMIT;
ext_ctrl_loc = SW.EXT_CTRL_LOC;
ext_run_enable = SW.EXT_RUN_ENABLE;
msw_b13 = SW.MSW_B13;
msw_b14 = SW.MSW_B14;
comm_err = SW.COMM_ERR;
